simulink model "simple_vehicle_dynamics_simulation_concept"  (R2022b)
settings: Solver=VariableStepAuto  StartTime=0.0  StopTime=50  RelTol=1e-3
libraries: slpidlib x1
settings Model: Creator=snazari  LastModifiedBy=ayush

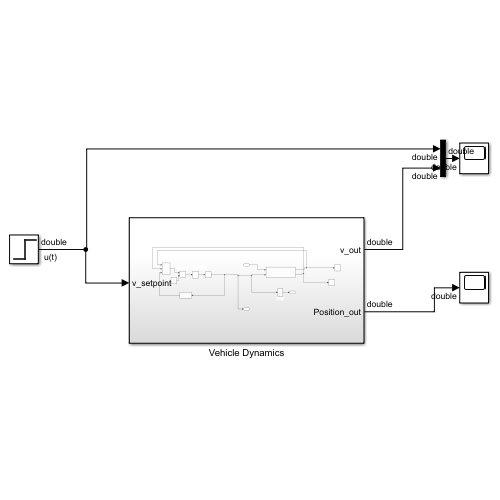
[thumbnail: Simulink's stored preview of the top-level diagram]
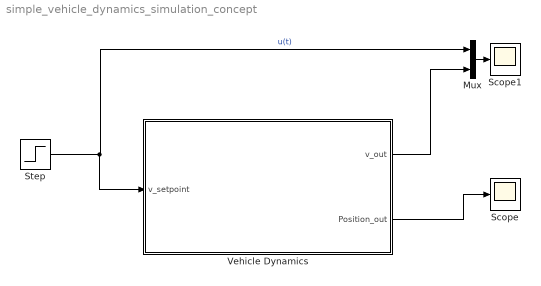
== system simple_vehicle_dynamics_simulation_concept ==
  Mux : Mux  Inputs=2
  Scope : Scope
  Scope1 : Scope
  Step : Step  After=35  SampleTime=0
  Vehicle Dynamics : Subsystem
  wires:
  Vehicle Dynamics/2(Position_out) -> Scope/1
  Step/1 -> Vehicle Dynamics/1(v_setpoint), Mux/1  "u(t)"
  Vehicle Dynamics/1(v_out) -> Mux/2
  Mux/1 -> Scope1/1

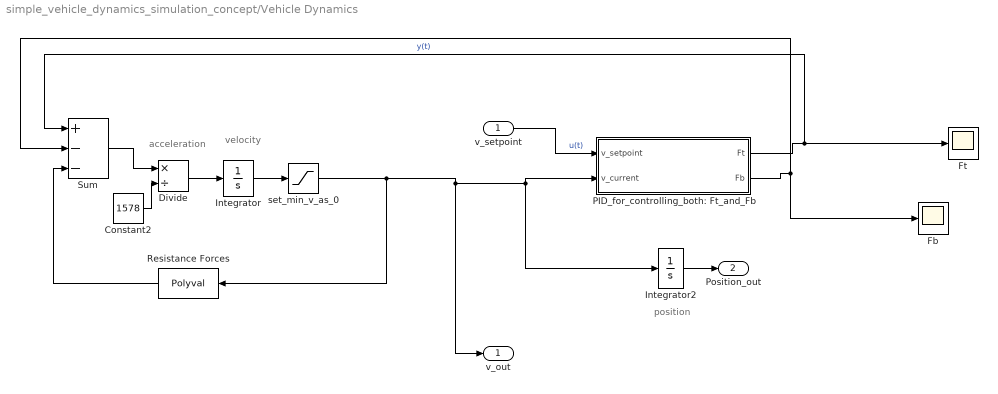
== system simple_vehicle_dynamics_simulation_concept/Vehicle Dynamics ==
  note: position
  note: acceleration
  note: velocity
  v_setpoint : Inport
  Constant2 : Constant  Value=1578
  Divide : Product  Inputs=*/
  Fb : Scope
  Ft : Scope
  Integrator : Integrator
  Integrator2 : Integrator
  PID_for_controlling_both: Ft_and_Fb : Subsystem
  Resistance Forces : Polyval  Coefs=[0.497 4.0349 97.33]
  Sum : Sum  Inputs=+--
  set_min_v_as_0 : Saturate  UpperLimit=3000  LowerLimit=0
  v_out : Outport
  Position_out : Outport  Port=2
  wires:
  v_setpoint/1 -> PID_for_controlling_both: Ft_and_Fb/1(v_setpoint)  "u(t)"
  Integrator/1 -> set_min_v_as_0/1
  Integrator2/1 -> Position_out/1
  Resistance Forces/1 -> Sum/3
  Sum/1 -> Divide/1
  Constant2/1 -> Divide/2
  Divide/1 -> Integrator/1
  PID_for_controlling_both: Ft_and_Fb/1(Ft) -> Ft/1, Sum/1  "y(t)"
  PID_for_controlling_both: Ft_and_Fb/2(Fb) -> Fb/1, Sum/2
  set_min_v_as_0/1 -> PID_for_controlling_both: Ft_and_Fb/2(v_current), Integrator2/1, v_out/1, Resistance Forces/1

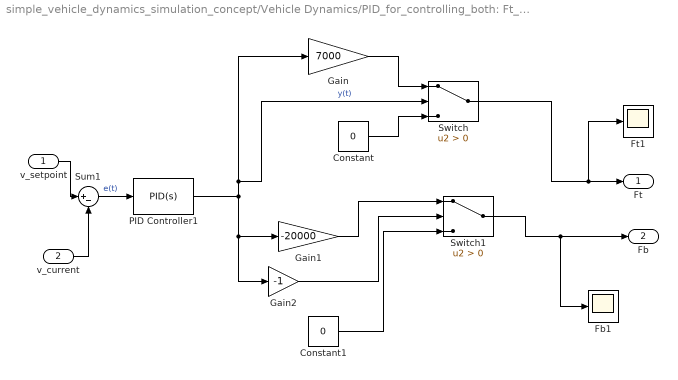
== system simple_vehicle_dynamics_simulation_concept/Vehicle Dynamics/PID_for_controlling_both: Ft_and_Fb ==
  v_setpoint : Inport
  v_current : Inport  Port=2
  Constant : Constant  Value=0
  Constant1 : Constant  Value=0
  Fb1 : Scope
  Ft1 : Scope
  Gain : Gain  Gain=7000
  Gain1 : Gain  Gain=-20000
  Gain2 : Gain  Gain=-1
  PID Controller1 : slpidlib/PID Controller  Controller=PID  Form=Parallel  TimeDomain=Continuous-time  UseExternalTs=off  SampleTime=-1  IntegratorMethod=Forward Euler  FilterMethod=Forward Euler  ControllerParametersSource=internal  P=38  I=2  UseKiTs=off  D=0  N=100  UseFilter=on  TunerSelectOption=Transfer Function Based (PID Tuner App)  InitialConditionSource=internal  InitialConditionForIntegrator=0  InitialConditionForFilter=0  DifferentiatorICPrevScaledInput=0  ExternalReset=none  TrackingMode=off  Kt=1  LimitOutput=on  SatLimitsSource=internal  UpperSaturationLimit=1  LowerSaturationLimit=-1  LinearizeAsGain=on  AntiWindupMode=none  Kb=1  LimitIntegrator=off  UpperIntegratorSaturationLimit=inf  LowerIntegratorSaturationLimit=-inf  POutMin=[]  POutMax=[]  IOutMin=[]  IOutMax=[]  DOutMin=[]  DOutMax=[]  NOutMin=[]  NOutMax=[]  SumOutMin=[]  SumOutMax=[]  SaturationOutMin=[]  SaturationOutMax=[]  PParamMin=[]  PParamMax=[]  IParamMin=[]  IParamMax=[]  DParamMin=[]  DParamMax=[]  NParamMin=[]  NParamMax=[]  KbParamMin=[]  KbParamMax=[]  KtParamMin=[]  KtParamMax=[]  KbOutMin=[]  KbOutMax=[]  KtOutMin=[]  KtOutMax=[]  IntegratorOutMin=[]  IntegratorOutMax=[]  FilterOutMin=[]  FilterOutMax=[]  SumI1OutMin=[]  SumI1OutMax=[]  SumI2OutMin=[]  SumI2OutMax=[]  SumI3OutMin=[]  SumI3OutMax=[]  SumI4OutMin=[]  SumI4OutMax=[]  SumDOutMin=[]  SumDOutMax=[]  DifferentiatorOutMin=[]  DifferentiatorOutMax=[]  FilterDiffOutCoefMin=[]  FilterDiffOutCoefMax=[]  ReciprocalOutMin=[]  ReciprocalOutMax=[]  SumDenOutMin=[]  SumDenOutMax=[]  SumNumOutMin=[]  SumNumOutMax=[]  DivideOutMin=[]  DivideOutMax=[]  UdiffTsProdOutMin=[]  UdiffTsProdOutMax=[]  NTsProdOutMin=[]  NTsProdOutMax=[]  UintegralTsProdOutMin=[]  UintegralTsProdOutMax=[]  UngainTsProdOutMin=[]  UngainTsProdOutMax=[]  ClampingZeroOutDataTypeStr=Inherit: Inherit via back propagation  ClampingZeroOutMin=[]  ClampingZeroOutMax=[]  FilterDenConstantOutDataTypeStr=Inherit: Inherit via back propagation  FilterDenConstantOutMin=[]  FilterDenConstantOutMax=[]  PCopyOutDataTypeStr=Inherit: Inherit via back propagation  PCopyOutMin=[]  PCopyOutMax=[]  NCopyOutDataTypeStr=Inherit: Inherit via back propagation  NCopyOutMin=[]  NCopyOutMax=[]  IntegratorContinuousStateAttributes=''  IntegratorStateMustResolveToSignalObject=off  IntegratorRTWStateStorageClass=Auto  FilterContinuousStateAttributes=''  FilterStateMustResolveToSignalObject=off  FilterRTWStateStorageClass=Auto  ParallelPVariant=InternalParameters  IdealPVariant=Disabled  IVariant=InternalParameters  DVariant=InternalParameters  IntegratorVariant=Continuous  SatVariant=Enabled  AWVariant=Passthrough  PCopyVariant=Disabled  TRVariant=Disabled  FdbkBlocksVariant=Forward  IdealPFdbkVariant=Disabled  SatFdbkVariant=Disabled  DerivativeFilterVariant=ContFilter  NVariant=InternalParameters  NCopyVariant=Disabled  FilterICVariant=InternalICsFilter  IntegratorICVariant=InternalICs  ExternalResetVariant=Disabled  TRSumVariant=Passthrough  SumFdbkVariant=Disabled  SumVariant=Sum_PID  TsampFilterVariant=InternalTs  TsampNgainVariant=Passthrough  TsampIntegralVariant=Passthrough  ExternalSaturationOutDataTypeStr=Inherit: Same as second input
  Sum1 : Sum  Inputs=|+-
  Switch : Switch  Criteria=u2 > Threshold  SaturateOnIntegerOverflow=off  InputSameDT=off
  Switch1 : Switch  Criteria=u2 > Threshold  SaturateOnIntegerOverflow=off  InputSameDT=off
  Ft : Outport
  Fb : Outport  Port=2
  wires:
  v_setpoint/1 -> Sum1/1
  PID Controller1/1 -> Gain2/1, Gain1/1, Gain/1, Switch/2  "y(t)"
  Sum1/1 -> PID Controller1/1  "e(t)"
  v_current/1 -> Sum1/2
  Switch1/1 -> Fb1/1, Fb/1
  Switch/1 -> Ft1/1, Ft/1
  Gain/1 -> Switch/1
  Constant/1 -> Switch/3
  Gain1/1 -> Switch1/1
  Constant1/1 -> Switch1/3
  Gain2/1 -> Switch1/2
